simulink model "CPU"  (R2024b)
settings: Solver=VariableStepAuto  StartTime=0.0  StopTime=100  RelTol=1e-3
libraries: simulink_extras x31
settings Model: NumberOfSteps=4  SnapshotBufferSize=30  SnapshotInterval=30  PacingRate=3  Creator=Reon Dsouze  LastModifiedBy=Reon Dsouze

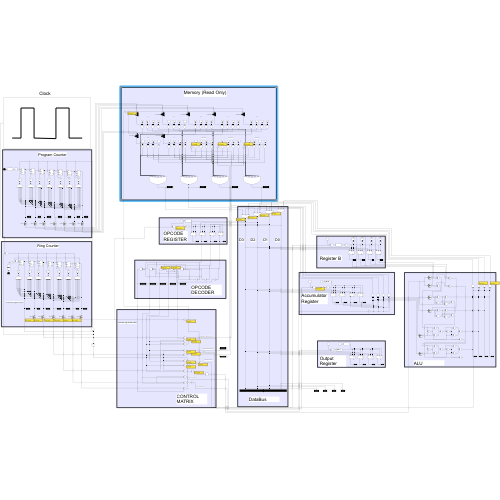
[thumbnail: Simulink's stored preview of the top-level diagram]
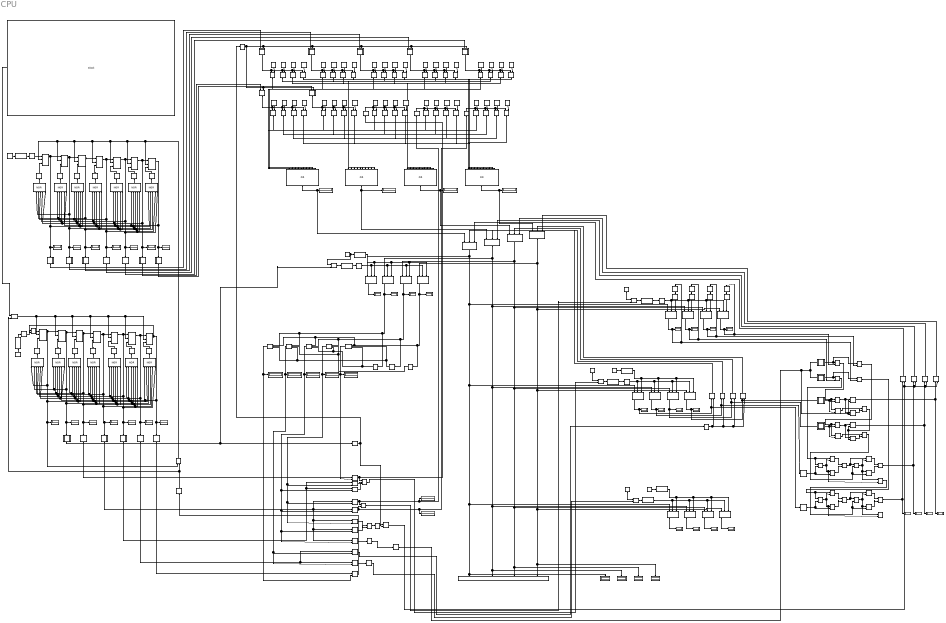
== system CPU ==
  note: Initial Value A
  note: D0
  note: Load A
  note: Ring Counter
  note: Clock
  note: Increment Program Counter
  note: CONTROL MATRIX
  note: enable A reg to data bus
  note: enable subtract
  note: enable sub to data bus from mem
  note: OPCODE DECODER
  note: enable ALU to data bus
  note: enable add to data bus from mem
  note: load A reg
  note: enable load a to data bus from mem
  note: load B reg
  note: halt
  note: Enable mmr to data bus
  note: Opcode reg latches data
  note: output reg latches data
  note: OPCODE
      | REGISTER
  note: Program Counter
  note: ADD
  note: ADD
  note: ADD
  note: SUB
  note: Output
  note: Halt
  note: DataBus
  note: D1
  note: D2
  note: D3
  note: Memory (Read Only)
  note: Accumulator
      | Register
  note: Output
      | Register
  note: Register B
  note: ALU
  note: Add Value B
  note: Sub Value B
  AND{,1,5..7,10..50,54..66} (59 alike) : Logic  IconShape=distinctive  AllPortsSameDT=off  OutDataTypeStr=boolean
  AND{8..9,51..53} (5 alike) : Logic  Inputs=3  IconShape=distinctive  AllPortsSameDT=off  OutDataTypeStr=boolean
  Bus Creator : BusCreator  Inputs=4
  Cast To Boolean{,1..8} (9 alike) : DataTypeConversion  OutDataTypeStr=boolean  SaturateOnIntegerOverflow=off  RndMeth=Floor
  Clock1 : simulink_extras/Flip Flops/Clock  period=2
  Constant{4..6,8..9,48,51,55,59,63..64,66,70,72,76,79,83..85} (19 alike) : Constant
  Constant{45..47,49..50,52..54,56..58,60..62,65,67..69,71,73..75,77..78,80..82} (27 alike) : Constant  Value=0
  D Flip-Flop{,1..29} (30 alike) : simulink_extras/Flip Flops/D Flip-Flop
  Delay{,1,6..7,12} (5 alike) : Delay  DelayLength=1
  Delay{2..5,8..11,119..129,132} (20 alike) : Delay
  Display{,1..48} (49 alike) : Display
  NAND{18..35,113..115,117..120,122..126,128} (31 alike) : Logic  Operator=NAND  IconShape=distinctive  AllPortsSameDT=off  OutDataTypeStr=boolean
  NAND121 : Logic  Operator=NAND  Inputs=3  IconShape=distinctive  AllPortsSameDT=off  OutDataTypeStr=boolean
  NOR{1..14} (14 alike) : Logic  Operator=NOR  Inputs=6  IconShape=distinctive  AllPortsSameDT=off  OutDataTypeStr=boolean
  NOT{,1..3,8..18,73} (16 alike) : Logic  Operator=NOT  IconShape=distinctive  AllPortsSameDT=off  OutDataTypeStr=boolean
  OR{10,12..14} (4 alike) : Logic  Operator=OR  Inputs=10  IconShape=distinctive  AllPortsSameDT=off  OutDataTypeStr=boolean
  OR11 : Logic  Operator=OR  IconShape=distinctive  AllPortsSameDT=off  OutDataTypeStr=boolean
  OR2 : Logic  Operator=OR  IconShape=distinctive  AllPortsSameDT=off  OutDataTypeStr=boolean
  OR3 : Logic  Operator=OR  IconShape=distinctive  AllPortsSameDT=off  OutDataTypeStr=boolean
  OR{6..9} (4 alike) : Logic  Operator=OR  Inputs=3  IconShape=distinctive  AllPortsSameDT=off  OutDataTypeStr=boolean
  Pulse Generator1 : DiscretePulseGenerator  PulseType=Time based  Period=1  PulseWidth=5
  Pulse Generator2 : DiscretePulseGenerator  PulseType=Time based  Period=1  PulseWidth=5
  Tri state buffer56 : Subsystem
      mask Display:
      | % Draw the triangle
      | patch([1 0 1], [0 0.5 1], [0 0 0])  % Left-pointing triangle
  Tri state buffer57 : Subsystem
      mask Display:
      | % Draw the triangle
      | patch([1 0 1], [0 0.5 1], [0 0 0])  % Left-pointing triangle
  Tri state buffer58 : Subsystem
      mask Display:
      | % Draw the triangle
      | patch([1 0 1], [0 0.5 1], [0 0 0])  % Left-pointing triangle
  Tri state buffer59 : Subsystem
      mask Display:
      | % Draw the triangle
      | patch([1 0 1], [0 0.5 1], [0 0 0])  % Left-pointing triangle
  Tri state buffer60 : Subsystem
      mask Display:
      | % Draw the triangle
      | patch([1 0 1], [0 0.5 1], [0 0 0])  % Left-pointing triangle
  Tri state buffer61 : Subsystem
      mask Display:
      | % Draw the triangle
      | patch([1 0 1], [0 0.5 1], [0 0 0])  % Left-pointing triangle
  Tri state buffer7 : Subsystem
      mask Display:
      | % Draw the triangle
      | patch([1 0 1], [0 0.5 1], [0 0 0])  % Left-pointing triangle
  XOR{8..15} (8 alike) : Logic  Operator=XOR  IconShape=distinctive  AllPortsSameDT=off  OutDataTypeStr=boolean
  buffer14 : Subsystem
      mask Display: patch([0 1 0], [0 0.5 1], [0.5 0.5 0.5]);  % This draws a triangle
  buffer16 : Subsystem
      mask Display: patch([0 1 0], [0 0.5 1], [0.5 0.5 0.5]);  % This draws a triangle
  buffer18 : Subsystem
      mask Display: patch([0 1 0], [0 0.5 1], [0.5 0.5 0.5]);  % This draws a triangle
  buffer20 : Subsystem
      mask Display: patch([0 1 0], [0 0.5 1], [0.5 0.5 0.5]);  % This draws a triangle
  buffer22 : Subsystem
      mask Display: patch([0 1 0], [0 0.5 1], [0.5 0.5 0.5]);  % This draws a triangle
  buffer23 : Subsystem
      mask Display: patch([0 1 0], [0 0.5 1], [0.5 0.5 0.5]);  % This draws a triangle
  buffer32 : Subsystem
      mask Display: patch([0 1 0], [0 0.5 1], [0.5 0.5 0.5]);  % This draws a triangle
  buffer33 : Subsystem
      mask Display: patch([0 1 0], [0 0.5 1], [0.5 0.5 0.5]);  % This draws a triangle
  buffer34 : Subsystem
      mask Display: patch([0 1 0], [0 0.5 1], [0.5 0.5 0.5]);  % This draws a triangle
  buffer35 : Subsystem
      mask Display: patch([0 1 0], [0 0.5 1], [0.5 0.5 0.5]);  % This draws a triangle
  buffer36 : Subsystem
      mask Display: patch([0 1 0], [0 0.5 1], [0.5 0.5 0.5]);  % This draws a triangle
  buffer37 : Subsystem
      mask Display: patch([0 1 0], [0 0.5 1], [0.5 0.5 0.5]);  % This draws a triangle
  buffer38 : Subsystem
      mask Display: patch([0 1 0], [0 0.5 1], [0.5 0.5 0.5]);  % This draws a triangle
  buffer40 : Subsystem
      mask Display: patch([0 1 0], [0 0.5 1], [0.5 0.5 0.5]);  % This draws a triangle
  buffer41 : Subsystem
      mask Display: patch([0 1 0], [0 0.5 1], [0.5 0.5 0.5]);  % This draws a triangle
  buffer42 : Subsystem
      mask Display: patch([0 1 0], [0 0.5 1], [0.5 0.5 0.5]);  % This draws a triangle
  buffer43 : Subsystem
      mask Display: patch([0 1 0], [0 0.5 1], [0.5 0.5 0.5]);  % This draws a triangle
  buffer44 : Subsystem
      mask Display: patch([0 1 0], [0 0.5 1], [0.5 0.5 0.5]);  % This draws a triangle
  buffer45 : Subsystem
      mask Display: patch([0 1 0], [0 0.5 1], [0.5 0.5 0.5]);  % This draws a triangle
  wires:
  buffer40/1(Out1) -> NAND120/1, NAND114/1
  NAND114/1 -> NAND121/2
  NAND123/1 -> NAND124/2, Display48/1, NOT18/1
  NAND128/1 -> NOT12/1
  buffer45/1(Out1) -> NAND125/1, NAND126/1, NAND115/1, NAND123/1, NAND122/1
  buffer42/1(Out1) -> NAND117/1, NAND118/1
  NAND122/1 -> Display12/1, NOT17/1, NAND124/1
  NAND118/1 -> NOT14/1
  NAND120/1 -> NAND121/3
  NAND115/1 -> NOT13/1
  NAND126/1 -> NAND128/2
  NAND125/1 -> NAND128/1
  Cast To Boolean1/1 -> Delay2/1
  OR11/1 -> D Flip-Flop4/1
  Pulse Generator1/1 -> Cast To Boolean1/1
  D Flip-Flop7/1 -> D Flip-Flop8/1, NOR5/2, NOR4/3, NOR10/4, NOR6/1, NOR9/5, NOR8/6, buffer45/1(In1), Display27/1
  Delay126/1 -> D Flip-Flop7/3
  Delay125/1 -> D Flip-Flop6/3
  Delay124/1 -> D Flip-Flop5/3
  Delay123/1 -> D Flip-Flop4/3
  D Flip-Flop6/1 -> D Flip-Flop7/1, NOR5/1, NOR10/3, NOR4/2, NOR9/4, NOR8/5, NOR7/6, Display26/1, buffer43/1(In1)
  D Flip-Flop5/1 -> D Flip-Flop6/1, NOR4/1, NOR10/2, NOR9/3, NOR8/4, NOR7/5, NOR6/6, Display25/1, buffer41/1(In1)
  D Flip-Flop8/1 -> NOR6/2, NOR5/3, NOR4/4, NOR10/5, NOR7/1, NOR9/6, buffer40/1(In1), Display28/1, D Flip-Flop9/1
  D Flip-Flop9/1 -> NOR4/5, NOR10/6, NOR5/4, NOR6/3, NOR7/2, NOR8/1, buffer42/1(In1), Display29/1, D Flip-Flop10/1
  D Flip-Flop10/1 -> OR11/1, NOR9/1, NOR7/3, NOR6/4, NOR5/5, NOR4/6, NOR8/2, buffer44/1(In1), Display30/1
  Delay127/1 -> D Flip-Flop8/3
  Delay128/1 -> D Flip-Flop9/3
  Delay129/1 -> D Flip-Flop10/3
  NOR4/1 -> Delay124/1
  NOR5/1 -> Delay125/1
  NOR6/1 -> Delay126/1
  NOR7/1 -> Delay127/1
  NOR8/1 -> Delay128/1
  NOR9/1 -> Delay129/1
  NOR10/1 -> Delay123/1
  NOR14/1 -> Delay132/1
  D Flip-Flop3/1 -> D Flip-Flop11/1, NOR1/2, NOR14/3, NOR13/4, NOR12/5, NOR11/6, Display21/1, buffer34/1(In1)
  D Flip-Flop11/1 -> D Flip-Flop12/1, NOR1/3, NOR2/2, NOR14/4, NOR13/5, NOR12/6, buffer36/1(In1), Display22/1
  D Flip-Flop12/1 -> D Flip-Flop13/1, NOR3/2, NOR2/3, NOR1/4, NOR14/5, NOR13/6, buffer38/1(In1), Display23/1
  Pulse Generator2/1 -> Cast To Boolean2/1
  NOR1/1 -> Delay4/1
  NOR11/1 -> Delay121/1
  NOR12/1 -> Delay120/1
  D Flip-Flop13/1 -> NOR11/2, NOR3/3, NOR2/4, NOR1/5, NOR14/6, buffer33/1(In1), Display31/1, D Flip-Flop14/1
  D Flip-Flop2/1 -> D Flip-Flop3/1, buffer32/1(In1), Display20/1, NOR14/2, NOR13/3, NOR12/4, NOR11/5, NOR3/6
  NOR3/1 -> Delay122/1
  Delay132/1 -> D Flip-Flop1/3
  Cast To Boolean2/1 -> Delay3/1
  NOR13/1 -> Delay119/1
  D Flip-Flop14/1 -> NOR2/5, NOR1/6, NOR3/4, NOR11/3, NOR12/2, buffer35/1(In1), Display32/1, D Flip-Flop1/1
  D Flip-Flop1/1 -> NOR12/3, NOR11/4, NOR3/5, NOR2/6, NOR13/2, buffer37/1(In1), Display33/1
  Delay119/1 -> D Flip-Flop14/3
  Delay120/1 -> D Flip-Flop13/3
  Delay121/1 -> D Flip-Flop12/3
  Delay122/1 -> D Flip-Flop11/3
  Constant45/1 -> AND10/2
  Constant46/1 -> AND11/2
  Constant47/1 -> AND12/2
  Constant48/1 -> AND13/2
  Constant52/1 -> AND17/2
  Constant51/1 -> AND16/2
  Constant50/1 -> AND15/2
  Constant49/1 -> AND14/2
  Constant53/1 -> AND18/2
  Constant54/1 -> AND19/2
  Constant55/1 -> AND20/2
  Constant56/1 -> AND21/2
  Constant60/1 -> AND25/2
  Constant59/1 -> AND24/2
  Constant58/1 -> AND23/2
  Constant57/1 -> AND22/2
  Constant84/1 -> AND49/2
  Constant83/1 -> AND48/2
  Constant82/1 -> AND47/2
  Constant81/1 -> AND46/2
  Constant77/1 -> AND42/2
  Constant78/1 -> AND43/2
  Constant79/1 -> AND44/2
  Constant80/1 -> AND45/2
  Constant76/1 -> AND41/2
  Constant75/1 -> AND40/2
  Constant74/1 -> AND39/2
  Constant73/1 -> AND38/2
  Constant68/1 -> AND33/2
  Constant67/1 -> AND32/2
  Constant66/1 -> AND31/2
  Constant65/1 -> AND30/2
  Tri state buffer7/1(Out1) -> AND12/1, AND13/1, AND11/1, AND10/1
  Tri state buffer56/1(Out1) -> AND17/1, AND16/1, AND15/1, AND14/1
  Tri state buffer58/1(Out1) -> AND21/1, AND20/1, AND19/1, AND18/1
  Tri state buffer57/1(Out1) -> AND25/1, AND24/1, AND23/1, AND22/1
  Tri state buffer61/1(Out1) -> AND33/1, AND32/1, AND31/1, AND30/1
  Tri state buffer59/1(Out1) -> AND26/1, AND27/1, AND28/1, AND29/1
  Constant61/1 -> AND26/2
  Constant62/1 -> AND27/2
  Constant63/1 -> AND28/2
  Constant64/1 -> AND29/2
  Tri state buffer60/1(Out1) -> AND34/1, AND35/1, AND36/1, AND37/1
  Constant69/1 -> AND34/2
  Constant70/1 -> AND35/2
  Constant71/1 -> AND36/2
  Constant72/1 -> AND37/2
  NOT73/1 -> Tri state buffer59/2(In2), Tri state buffer57/2(In2), Tri state buffer58/2(In2), Tri state buffer56/2(In2), Tri state buffer7/2(In2), Tri state buffer60/2(In2), Tri state buffer61/2(In2)
  buffer32/1(Out1) -> Tri state buffer7/1(In1)
  buffer34/1(Out1) -> Tri state buffer56/1(In1)
  buffer36/1(Out1) -> Tri state buffer58/1(In1)
  buffer38/1(Out1) -> Tri state buffer57/1(In1)
  buffer33/1(Out1) -> Tri state buffer59/1(In1)
  buffer35/1(Out1) -> Tri state buffer61/1(In1)
  buffer37/1(Out1) -> Tri state buffer60/1(In1)
  AND30/1 -> OR10/6
  AND10/1 -> OR10/1
  AND14/1 -> OR10/2
  AND18/1 -> OR10/3
  AND22/1 -> OR10/4
  AND26/1 -> OR10/5
  AND34/1 -> OR10/7
  AND38/1 -> OR10/8
  AND42/1 -> OR10/9
  AND46/1 -> OR10/10
  AND11/1 -> OR12/1
  AND15/1 -> OR12/2
  AND19/1 -> OR12/3
  AND23/1 -> OR12/4
  AND27/1 -> OR12/5
  AND31/1 -> OR12/6
  AND35/1 -> OR12/7
  AND39/1 -> OR12/8
  AND43/1 -> OR12/9
  AND47/1 -> OR12/10
  AND12/1 -> OR13/1
  AND16/1 -> OR13/2
  AND20/1 -> OR13/3
  AND24/1 -> OR13/4
  AND28/1 -> OR13/5
  AND32/1 -> OR13/6
  AND36/1 -> OR13/7
  AND44/1 -> OR13/8
  AND48/1 -> OR13/10
  AND40/1 -> OR13/9
  AND13/1 -> OR14/1
  AND17/1 -> OR14/2
  AND21/1 -> OR14/3
  AND25/1 -> OR14/4
  AND29/1 -> OR14/5
  AND33/1 -> OR14/6
  AND37/1 -> OR14/7
  AND41/1 -> OR14/8
  AND45/1 -> OR14/9
  AND49/1 -> OR14/10
  OR10/1 -> OR6/1, Display13/1
  OR12/1 -> OR7/1, Display14/1
  OR13/1 -> OR8/1, Display15/1
  OR14/1 -> OR9/1, Display16/1
  AND50/1 -> Cast To Boolean/1
  D Flip-Flop/1 -> Display17/1
  D Flip-Flop16/1 -> AND53/2, AND52/1, NOT8/1, Display18/1
  D Flip-Flop18/1 -> AND51/2, AND9/1, NOT9/1, Display19/1
  D Flip-Flop19/1 -> AND51/1, AND53/1, AND8/1, NOT16/1, Display34/1
  Cast To Boolean3/1 -> D Flip-Flop19/3, D Flip-Flop18/3, D Flip-Flop16/3, D Flip-Flop/3
  Constant85/1 -> AND50/1, Cast To Boolean3/1
  NOT9/1 -> AND53/3, AND52/3, AND8/2
  NOT8/1 -> AND51/3, AND9/3, AND8/3
  NOT16/1 -> AND52/2, AND9/2
  AND53/1 -> NAND119/2, Display35/1
  AND52/1 -> NAND117/2, NAND118/2, Display36/1
  AND51/1 -> NAND115/2, NAND126/2, NAND123/2, NAND120/2, Display37/1
  AND8/1 -> Display39/1, NAND113/2
  Clock1/1 -> AND54/1
  Cast To Boolean/1 -> Delay/1
  AND54/1 -> D Flip-Flop10/2, D Flip-Flop9/2, D Flip-Flop8/2, D Flip-Flop7/2, D Flip-Flop6/2, D Flip-Flop5/2, D Flip-Flop4/2
  buffer44/1(Out1) -> NAND119/1
  Delay2/1 -> OR11/2
  Delay3/1 -> D Flip-Flop2/1
  D Flip-Flop21/1 -> buffer18/1(In1), AND60/1, Display7/1
  Cast To Boolean5/1 -> D Flip-Flop21/3, D Flip-Flop20/3, D Flip-Flop17/3, D Flip-Flop15/3
  Cast To Boolean4/1 -> Delay7/1
  D Flip-Flop17/1 -> AND58/1, buffer22/1(In1), Display5/1
  D Flip-Flop23/1 -> Display41/1
  Cast To Boolean6/1 -> D Flip-Flop25/2, D Flip-Flop24/2, D Flip-Flop23/2, D Flip-Flop22/2
  D Flip-Flop24/1 -> Display42/1
  Cast To Boolean7/1 -> D Flip-Flop22/3, D Flip-Flop23/3, D Flip-Flop24/3, D Flip-Flop25/3
  D Flip-Flop22/1 -> Display40/1
  AND56/1 -> Cast To Boolean6/1
  D Flip-Flop25/1 -> Display43/1
  Constant4/1 -> Cast To Boolean5/1
  Constant5/1 -> Cast To Boolean7/1
  AND57/1 -> OR6/2
  AND58/1 -> OR7/2
  AND59/1 -> OR8/2
  AND60/1 -> OR9/2
  NOT10/1 -> AND59/2, AND60/2, AND58/2, AND57/2
  Constant6/1 -> AND55/1
  AND55/1 -> Cast To Boolean4/1
  OR6/1 -> Display8/1, Bus Creator/1, D Flip-Flop22/1, D Flip-Flop15/1, D Flip-Flop26/1, D Flip-Flop/1
  OR7/1 -> D Flip-Flop23/1, Bus Creator/2, Display9/1, D Flip-Flop17/1, D Flip-Flop27/1, D Flip-Flop16/1
  OR8/1 -> D Flip-Flop24/1, Bus Creator/3, Display10/1, D Flip-Flop20/1, D Flip-Flop28/1, D Flip-Flop18/1
  OR9/1 -> D Flip-Flop25/1, Bus Creator/4, Display11/1, D Flip-Flop21/1, D Flip-Flop29/1, D Flip-Flop19/1
  D Flip-Flop29/1 -> Delay11/1, XOR8/2, Display47/1
  AND61/1 -> Cast To Boolean8/1
  D Flip-Flop26/1 -> Delay8/1, XOR11/2, Display44/1
  D Flip-Flop28/1 -> Delay10/1, XOR10/2, Display46/1
  D Flip-Flop27/1 -> Delay9/1, XOR9/2, Display45/1
  Constant8/1 -> AND56/1
  NOT14/1 -> AND56/2
  Constant9/1 -> AND61/1
  NAND117/1 -> NOT10/1
  NOT11/1 -> AND38/1, AND39/1, AND40/1, AND41/1
  NOT17/1 -> AND42/1, AND43/1, AND45/1, AND44/1
  NOT18/1 -> AND46/1, AND49/1, AND48/1, AND47/1
  buffer14/1(Out1) -> XOR10/1, XOR8/1
  buffer16/1(Out1) -> XOR11/1, XOR9/1
  NOT13/1 -> Delay12/1
  buffer18/1(Out1) -> XOR12/2, AND5/2
  XOR8/1 -> XOR12/1, AND5/1
  XOR12/1 -> AND6/1, XOR13/1
  AND5/1 -> OR2/1
  AND6/1 -> OR2/2
  AND62/1 -> OR3/2
  AND7/1 -> OR3/1
  XOR14/1 -> XOR15/1, AND62/1
  XOR10/1 -> AND7/1, XOR14/1
  buffer20/1(Out1) -> AND7/2, XOR14/2
  OR2/1 -> XOR15/2, AND62/2
  D Flip-Flop20/1 -> Display6/1, buffer20/1(In1), AND59/1
  NAND18/1 -> NAND26/2, NAND20/1, NAND19/2
  NAND19/1 -> NAND21/1
  NAND20/1 -> NAND21/2
  NAND24/1 -> NAND25/2
  NAND23/1 -> NAND25/1
  NAND22/1 -> NAND23/2, NAND24/1, NAND26/1
  NAND21/1 -> NAND22/1, NAND23/1
  OR3/1 -> NAND24/2, NAND22/2
  buffer22/1(Out1) -> NAND18/2, NAND20/2
  XOR9/1 -> NAND19/1, NAND18/1
  XOR11/1 -> NAND27/1, NAND28/1
  buffer23/1(Out1) -> NAND29/2, NAND27/2
  NAND26/1 -> NAND31/2, NAND33/2
  NAND30/1 -> NAND32/1, NAND31/1
  NAND31/1 -> NAND35/1, NAND33/1, NAND32/2
  NAND32/1 -> NAND34/1
  NAND33/1 -> NAND34/2
  NAND29/1 -> NAND30/2
  NAND28/1 -> NAND30/1
  NAND27/1 -> NAND28/2, NAND29/1, NAND35/2
  D Flip-Flop15/1 -> buffer23/1(In1), AND57/1, Display4/1
  XOR13/1 -> Display3/1, AND66/1
  XOR15/1 -> Display2/1, AND65/1
  NAND25/1 -> Display1/1, AND64/1
  NAND34/1 -> Display/1, AND63/1
  AND63/1 -> OR6/3
  AND64/1 -> OR7/3
  AND65/1 -> OR8/3
  AND66/1 -> OR9/3
  buffer43/1(Out1) -> NAND113/1
  Delay4/1 -> D Flip-Flop2/3
  NOR2/1 -> Delay5/1
  Delay5/1 -> D Flip-Flop3/3
  AND/1 -> AND63/2, AND64/2, AND65/2, AND66/2
  AND9/1 -> NAND114/2, NAND125/2, NAND122/2, Display38/1
  NAND124/1 -> AND61/2
  Cast To Boolean8/1 -> Delay6/1
  NAND121/1 -> AND55/2
  NOT15/1 -> AND/1, NOT73/1
  buffer41/1(Out1) -> NOT15/1, AND50/2
  NAND113/1 -> NOT11/1, NAND121/1
  Delay/1 -> D Flip-Flop/2, D Flip-Flop16/2, D Flip-Flop18/2, D Flip-Flop19/2
  Delay6/1 -> D Flip-Flop26/2, D Flip-Flop27/2, D Flip-Flop28/2, D Flip-Flop29/2
  Delay7/1 -> D Flip-Flop15/2, D Flip-Flop17/2, D Flip-Flop20/2, D Flip-Flop21/2
  NOT/1 -> D Flip-Flop26/3
  Delay8/1 -> NOT/1
  Delay9/1 -> NOT1/1
  NOT1/1 -> D Flip-Flop27/3
  NOT2/1 -> D Flip-Flop28/3
  Delay10/1 -> NOT2/1
  Delay11/1 -> NOT3/1
  NOT3/1 -> D Flip-Flop29/3
  Delay12/1 -> buffer16/1(In1), buffer14/1(In1), XOR13/2, AND6/2
  NOT12/1 -> AND/2
  AND1/1 -> D Flip-Flop2/2, D Flip-Flop3/2, D Flip-Flop11/2, D Flip-Flop12/2, D Flip-Flop13/2, D Flip-Flop14/2, D Flip-Flop1/2
  NAND119/1 -> Delay1/1
  Delay1/1 -> AND54/2, AND1/2
  D Flip-Flop4/1 -> AND1/1, Display24/1, NOR9/2, NOR8/3, NOR7/4, NOR6/5, NOR5/6, NOR10/1, D Flip-Flop5/1

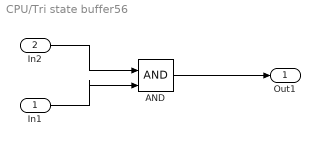
== system CPU/Tri state buffer56 ==
  In1 : Inport
  In2 : Inport  Port=2
  AND : Logic  IconShape=distinctive  AllPortsSameDT=off  OutDataTypeStr=boolean
  Out1 : Outport
  wires:
  In1/1 -> AND/2
  In2/1 -> AND/1
  AND/1 -> Out1/1

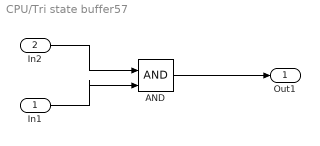
== system CPU/Tri state buffer57 ==
  In1 : Inport
  In2 : Inport  Port=2
  AND : Logic  IconShape=distinctive  AllPortsSameDT=off  OutDataTypeStr=boolean
  Out1 : Outport
  wires:
  AND/1 -> Out1/1
  In2/1 -> AND/1
  In1/1 -> AND/2

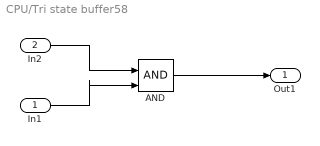
== system CPU/Tri state buffer58 ==
  In1 : Inport
  In2 : Inport  Port=2
  AND : Logic  IconShape=distinctive  AllPortsSameDT=off  OutDataTypeStr=boolean
  Out1 : Outport
  wires:
  In1/1 -> AND/2
  In2/1 -> AND/1
  AND/1 -> Out1/1

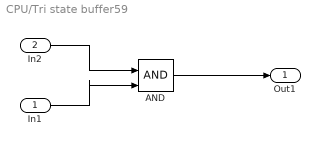
== system CPU/Tri state buffer59 ==
  In1 : Inport
  In2 : Inport  Port=2
  AND : Logic  IconShape=distinctive  AllPortsSameDT=off  OutDataTypeStr=boolean
  Out1 : Outport
  wires:
  In1/1 -> AND/2
  In2/1 -> AND/1
  AND/1 -> Out1/1

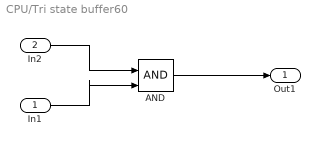
== system CPU/Tri state buffer60 ==
  In1 : Inport
  In2 : Inport  Port=2
  AND : Logic  IconShape=distinctive  AllPortsSameDT=off  OutDataTypeStr=boolean
  Out1 : Outport
  wires:
  AND/1 -> Out1/1
  In2/1 -> AND/1
  In1/1 -> AND/2

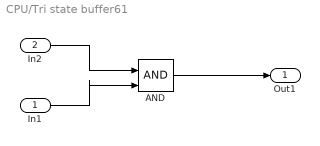
== system CPU/Tri state buffer61 ==
  In1 : Inport
  In2 : Inport  Port=2
  AND : Logic  IconShape=distinctive  AllPortsSameDT=off  OutDataTypeStr=boolean
  Out1 : Outport
  wires:
  In1/1 -> AND/2
  In2/1 -> AND/1
  AND/1 -> Out1/1

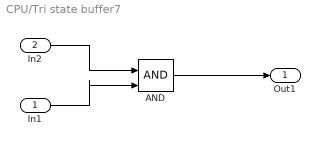
== system CPU/Tri state buffer7 ==
  In1 : Inport
  In2 : Inport  Port=2
  AND : Logic  IconShape=distinctive  AllPortsSameDT=off  OutDataTypeStr=boolean
  Out1 : Outport
  wires:
  AND/1 -> Out1/1
  In2/1 -> AND/1
  In1/1 -> AND/2

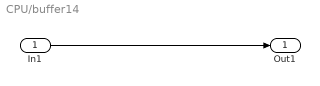
== system CPU/buffer14 ==
  In1 : Inport
  Out1 : Outport
  wires:
  In1/1 -> Out1/1

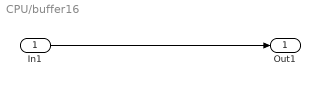
== system CPU/buffer16 ==
  In1 : Inport
  Out1 : Outport
  wires:
  In1/1 -> Out1/1

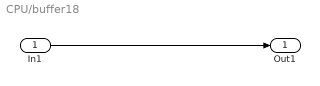
== system CPU/buffer18 ==
  In1 : Inport
  Out1 : Outport
  wires:
  In1/1 -> Out1/1

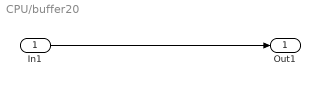
== system CPU/buffer20 ==
  In1 : Inport
  Out1 : Outport
  wires:
  In1/1 -> Out1/1

== system CPU/buffer22 ==
  In1 : Inport
  Out1 : Outport
  wires:
  In1/1 -> Out1/1

== system CPU/buffer23 ==
  In1 : Inport
  Out1 : Outport
  wires:
  In1/1 -> Out1/1

== system CPU/buffer32 ==
  In1 : Inport
  Out1 : Outport
  wires:
  In1/1 -> Out1/1

== system CPU/buffer33 ==
  In1 : Inport
  Out1 : Outport
  wires:
  In1/1 -> Out1/1

== system CPU/buffer34 ==
  In1 : Inport
  Out1 : Outport
  wires:
  In1/1 -> Out1/1

== system CPU/buffer35 ==
  In1 : Inport
  Out1 : Outport
  wires:
  In1/1 -> Out1/1

== system CPU/buffer36 ==
  In1 : Inport
  Out1 : Outport
  wires:
  In1/1 -> Out1/1

== system CPU/buffer37 ==
  In1 : Inport
  Out1 : Outport
  wires:
  In1/1 -> Out1/1

== system CPU/buffer38 ==
  In1 : Inport
  Out1 : Outport
  wires:
  In1/1 -> Out1/1

== system CPU/buffer40 ==
  In1 : Inport
  Out1 : Outport
  wires:
  In1/1 -> Out1/1

== system CPU/buffer41 ==
  In1 : Inport
  Out1 : Outport
  wires:
  In1/1 -> Out1/1

== system CPU/buffer42 ==
  In1 : Inport
  Out1 : Outport
  wires:
  In1/1 -> Out1/1

== system CPU/buffer43 ==
  In1 : Inport
  Out1 : Outport
  wires:
  In1/1 -> Out1/1

== system CPU/buffer44 ==
  In1 : Inport
  Out1 : Outport
  wires:
  In1/1 -> Out1/1

== system CPU/buffer45 ==
  In1 : Inport
  Out1 : Outport
  wires:
  In1/1 -> Out1/1
